simulink model "Area_TestModel"  (R2014a)
settings: Solver=ode45  StartTime=0.0  StopTime=10.0  RelTol=1e-3
libraries: rocket_drag_library x2
settings Model: Creator=scorpii  LastModifiedBy=scorpii

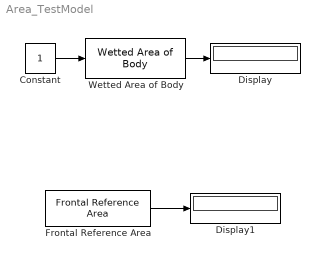
== system Area_TestModel ==
  Constant : Constant
  Display : Display
  Display1 : Display
  Frontal Reference Area : rocket_drag_library/Frontal Reference Area
      link override AreaReferenceFrontal/AreaReferenceFrontal: MATLABFcn=AreaReferenceFrontal
  Wetted Area of Body : rocket_drag_library/Wetted Area of Body
  wires:
  Wetted Area of Body/1 -> Display/1
  Frontal Reference Area/1 -> Display1/1
  Constant/1 -> Wetted Area of Body/1
